simulink model "Base_Model"  (R2023b)
settings: Solver=VariableStepAuto  StartTime=0.0  StopTime=120  RelTol=1e-3
undefined symbols (not defined in the file): D1, D2, I
libraries: simulink x3, mcbcontrolslib x2
settings Model: Creator=markzhuang  LastModifiedBy=markzhuang

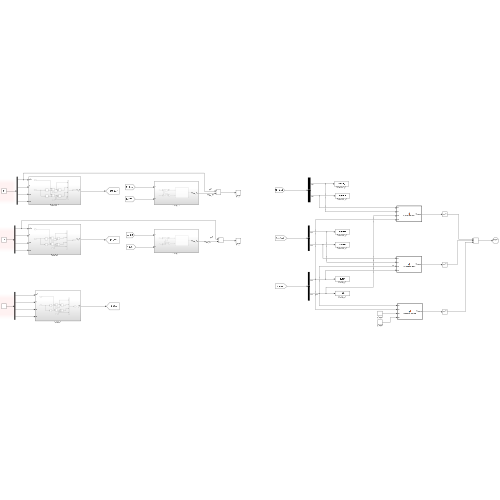
[thumbnail: Simulink's stored preview of the top-level diagram]
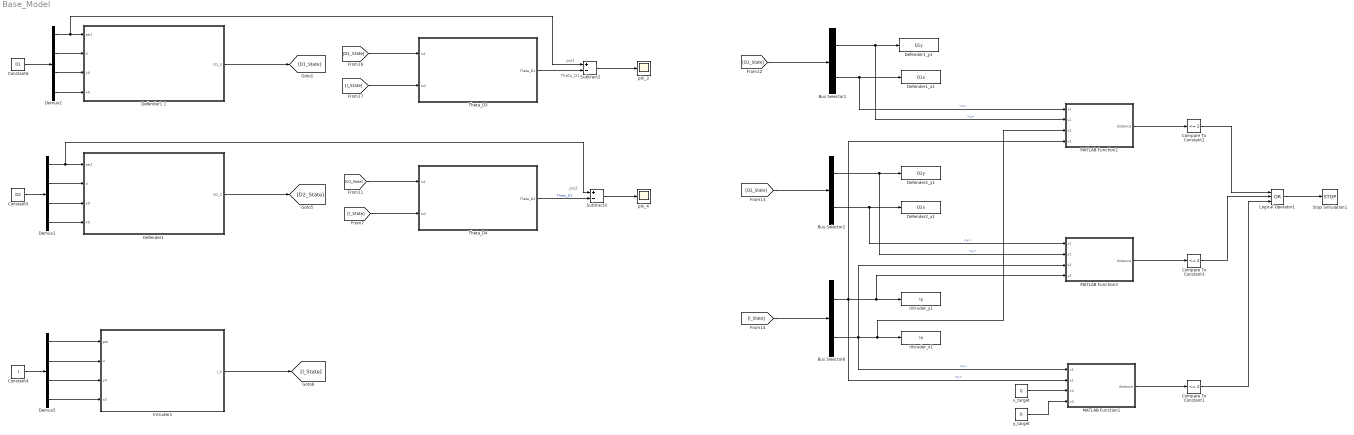
== system Base_Model ==
  note: psi2
  note: psi1
  note: Theta_D1
  Bus Selector1 : BusSelector  OutputSignals=y,x
  Bus Selector2 : BusSelector  OutputSignals=y,x
  Bus Selector6 : BusSelector  OutputSignals=y,x
  Compare To Constant1 : simulink/Logic and Bit Operations/Compare To Constant  relop=<=  const=2  OutDataTypeStr=boolean
  Compare To Constant2 : simulink/Logic and Bit Operations/Compare To Constant  relop=<=  const=2  OutDataTypeStr=boolean
  Compare To Constant3 : simulink/Logic and Bit Operations/Compare To Constant  relop=<=  const=2  OutDataTypeStr=boolean
  Constant4 : Constant  Value=I  VectorParams1D=off
  Constant5 : Constant  Value=D2  VectorParams1D=off
  Constant6 : Constant  Value=D1  VectorParams1D=off
  Defender1 : Subsystem
  Defender1 1 : Subsystem
  Defender1_x1 : ToWorkspace  VariableName=D1x  SaveFormat=Timeseries  SampleTime=-1
  Defender1_y1 : ToWorkspace  VariableName=D1y  SaveFormat=Timeseries  SampleTime=-1
  Defender2_x1 : ToWorkspace  VariableName=D2x  SaveFormat=Timeseries  SampleTime=-1
  Defender2_y1 : ToWorkspace  VariableName=D2y  SaveFormat=Timeseries  SampleTime=-1
  Demux1 : Demux
  Demux2 : Demux
  Demux5 : Demux
  Intruder1 : Subsystem
  Intruder_x1 : ToWorkspace  VariableName=Ix  SaveFormat=Timeseries  SampleTime=-1
  Intruder_y1 : ToWorkspace  VariableName=Iy  SaveFormat=Timeseries  SampleTime=-1
  Logical Operator1 : Logic  Operator=OR  Inputs=3  AllPortsSameDT=off  OutDataTypeStr=boolean
  MATLAB Function1 : MATLAB Function  TreatAsAtomicUnit=on
  MATLAB Function2 : MATLAB Function  TreatAsAtomicUnit=on
  MATLAB Function3 : MATLAB Function  TreatAsAtomicUnit=on
  Stop Simulation1 : Stop
  Subtract2 : Sum  Inputs=+-
  Subtract3 : Sum  Inputs=+-
  Theta_D3 : Subsystem
  Theta_D4 : Subsystem
  phi_3 : Scope
  phi_4 : Scope
  x_target : Constant  Value=0
  y_target : Constant  Value=0
  wires:
  Bus Selector1/2 -> MATLAB Function2/1(x1), Defender1_x1/1  "<x>"
  Demux5/3 -> Intruder1/3(y0)
  Demux5/4 -> Intruder1/4(x0)
  [D2_State] -> Theta_D4/1(In1)
  [D1_State] -> Theta_D3/1(In1)
  Bus Selector1/1 -> MATLAB Function2/2(y1), Defender1_y1/1  "<y>"
  Demux2/2 -> Defender1 1/2(V)
  y_target/1 -> MATLAB Function1/4(y2)
  Defender1 1/1(D1_S) -> [D1_State]
  Demux5/2 -> Intruder1/2(V)
  Demux2/3 -> Defender1 1/3(y0)
  Bus Selector6/1 -> MATLAB Function1/2(y1), MATLAB Function2/4(y2), MATLAB Function3/4(y2), Intruder_y1/1  "<y>"
  Demux5/1 -> Intruder1/1(psiI)
  Defender1/1(D2_S) -> [D2_State]
  [I_State] -> Theta_D3/2(In2)
  [I_State] -> Theta_D4/2(In2)
  Demux1/4 -> Defender1/4(x0)
  Constant6/1 -> Demux2/1
  MATLAB Function1/1(distance) -> Compare To Constant1/1
  Constant4/1 -> Demux5/1
  Demux1/2 -> Defender1/2(V)
  [D2_State] -> Bus Selector2/1
  Subtract2/1 -> phi_3/1
  MATLAB Function2/1(distance) -> Compare To Constant2/1
  MATLAB Function3/1(distance) -> Compare To Constant3/1
  Compare To Constant3/1 -> Logical Operator1/2
  Bus Selector2/1 -> MATLAB Function3/2(y1), Defender2_y1/1  "<y>"
  Demux1/3 -> Defender1/3(y0)
  Compare To Constant1/1 -> Logical Operator1/3
  Subtract3/1 -> phi_4/1
  Bus Selector2/2 -> MATLAB Function3/1(x1), Defender2_x1/1  "<x>"
  Demux2/4 -> Defender1 1/4(x0)
  Bus Selector6/2 -> MATLAB Function3/3(x2), MATLAB Function1/1(x1), MATLAB Function2/3(x2), Intruder_x1/1  "<x>"
  x_target/1 -> MATLAB Function1/3(x2)
  [D1_State] -> Bus Selector1/1
  Theta_D3/1(Theta_D1) -> Subtract2/2
  Logical Operator1/1 -> Stop Simulation1/1
  Compare To Constant2/1 -> Logical Operator1/1
  Intruder1/1(I_S) -> [I_State]
  Constant5/1 -> Demux1/1
  [I_State] -> Bus Selector6/1
  Theta_D4/1(Theta_D2) -> Subtract3/2  "Theta_D2"
  Demux2/1 -> Subtract2/1, Defender1 1/1(psi1)
  Demux1/1 -> Subtract3/1, Defender1/1(psi2)

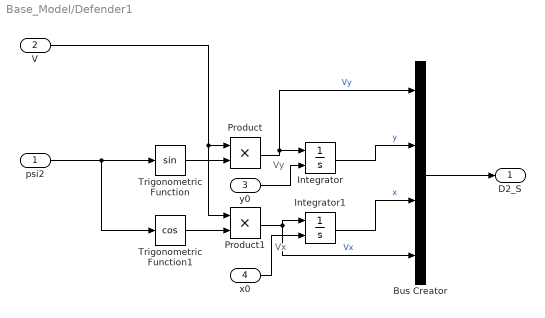
== system Base_Model/Defender1 ==
  note: Vx
  note: Vy
  psi2 : Inport
  V : Inport  Port=2
  y0 : Inport  Port=3
  x0 : Inport  Port=4
  Bus Creator : BusCreator  Inputs=4
  Integrator : Integrator  InitialConditionSource=external
  Integrator1 : Integrator  InitialConditionSource=external
  Product : Product
  Product1 : Product
  Trigonometric Function : Trigonometry
  Trigonometric Function1 : Trigonometry  Operator=cos
  D2_S : Outport
  wires:
  Trigonometric Function/1 -> Product/2
  Product/1 -> Bus Creator/1, Integrator/1  "Vy"
  psi2/1 -> Trigonometric Function1/1, Trigonometric Function/1
  Product1/1 -> Bus Creator/4, Integrator1/1  "Vx"
  V/1 -> Product1/1, Product/1
  Trigonometric Function1/1 -> Product1/2
  Integrator/1 -> Bus Creator/2  "y"
  Integrator1/1 -> Bus Creator/3  "x"
  y0/1 -> Integrator/2
  x0/1 -> Integrator1/2
  Bus Creator/1 -> D2_S/1

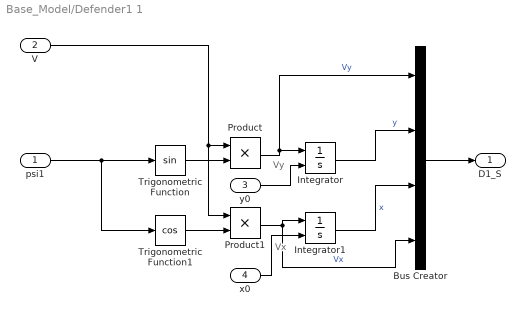
== system Base_Model/Defender1 1 ==
  note: Vx
  note: Vy
  psi1 : Inport
  V : Inport  Port=2
  y0 : Inport  Port=3
  x0 : Inport  Port=4
  Bus Creator : BusCreator  Inputs=4
  Integrator : Integrator  InitialConditionSource=external
  Integrator1 : Integrator  InitialConditionSource=external
  Product : Product
  Product1 : Product
  Trigonometric Function : Trigonometry
  Trigonometric Function1 : Trigonometry  Operator=cos
  D1_S : Outport
  wires:
  Trigonometric Function/1 -> Product/2
  psi1/1 -> Trigonometric Function1/1, Trigonometric Function/1
  Product1/1 -> Bus Creator/4, Integrator1/1  "Vx"
  V/1 -> Product1/1, Product/1
  Trigonometric Function1/1 -> Product1/2
  y0/1 -> Integrator/2
  x0/1 -> Integrator1/2
  Product/1 -> Bus Creator/1, Integrator/1  "Vy"
  Integrator/1 -> Bus Creator/2  "y"
  Integrator1/1 -> Bus Creator/3  "x"
  Bus Creator/1 -> D1_S/1

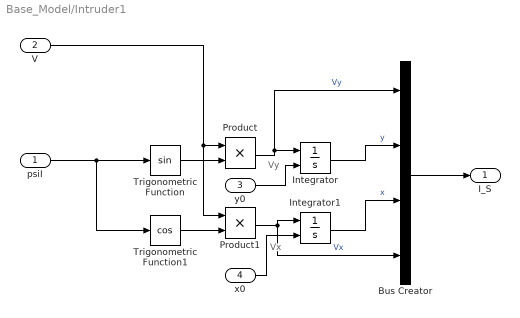
== system Base_Model/Intruder1 ==
  note: Vx
  note: Vy
  psiI : Inport
  V : Inport  Port=2
  y0 : Inport  Port=3
  x0 : Inport  Port=4
  Bus Creator : BusCreator  Inputs=4
  Integrator : Integrator  InitialConditionSource=external
  Integrator1 : Integrator  InitialConditionSource=external
  Product : Product
  Product1 : Product
  Trigonometric Function : Trigonometry
  Trigonometric Function1 : Trigonometry  Operator=cos
  I_S : Outport
  wires:
  Trigonometric Function/1 -> Product/2
  Product/1 -> Bus Creator/1, Integrator/1  "Vy"
  psiI/1 -> Trigonometric Function1/1, Trigonometric Function/1
  Product1/1 -> Bus Creator/4, Integrator1/1  "Vx"
  V/1 -> Product1/1, Product/1
  Trigonometric Function1/1 -> Product1/2
  Integrator/1 -> Bus Creator/2  "y"
  Integrator1/1 -> Bus Creator/3  "x"
  y0/1 -> Integrator/2
  x0/1 -> Integrator1/2
  Bus Creator/1 -> I_S/1

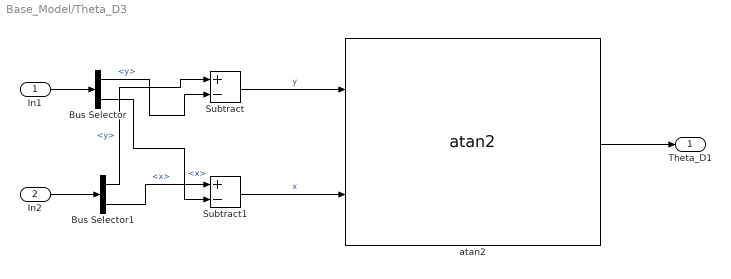
== system Base_Model/Theta_D3 ==
  In1 : Inport
  In2 : Inport  Port=2
  Bus Selector : BusSelector  OutputSignals=y,x
  Bus Selector1 : BusSelector  OutputSignals=y,x
  Subtract : Sum  Inputs=+-
  Subtract1 : Sum  Inputs=+-
  atan2 : mcbcontrolslib/atan2  ApproximationMethod=None  NumberOfIterations=11  NumberOfDataPoints=16  InterpMethod=Flat  outputUnit=Radians  TableDataTypeStr=Inherit: Inherit via input
      settings: LibrarySourceBlock=mcblib/Controls/Math Transforms/atan2
  Theta_D1 : Outport
  wires:
  In1/1 -> Bus Selector/1
  In2/1 -> Bus Selector1/1
  Bus Selector1/1 -> Subtract/1  "<y>"
  Bus Selector/1 -> Subtract/2  "<y>"
  Bus Selector1/2 -> Subtract1/1  "<x>"
  Bus Selector/2 -> Subtract1/2  "<x>"
  Subtract/1 -> atan2/1  "y"
  Subtract1/1 -> atan2/2  "x"
  atan2/1 -> Theta_D1/1

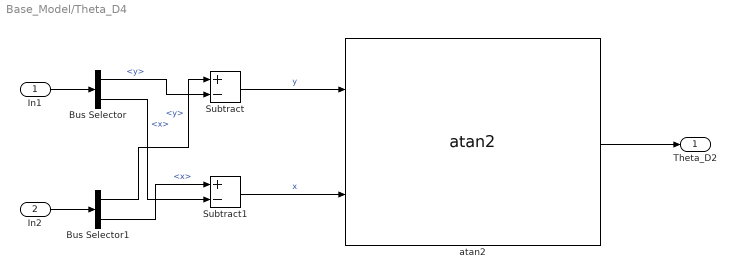
== system Base_Model/Theta_D4 ==
  In1 : Inport
  In2 : Inport  Port=2
  Bus Selector : BusSelector  OutputSignals=y,x
  Bus Selector1 : BusSelector  OutputSignals=y,x
  Subtract : Sum  Inputs=+-
  Subtract1 : Sum  Inputs=+-
  atan2 : mcbcontrolslib/atan2  ApproximationMethod=None  NumberOfIterations=11  NumberOfDataPoints=16  InterpMethod=Flat  outputUnit=Radians  TableDataTypeStr=Inherit: Inherit via input
      settings: LibrarySourceBlock=mcblib/Controls/Math Transforms/atan2
  Theta_D2 : Outport
  wires:
  In1/1 -> Bus Selector/1
  In2/1 -> Bus Selector1/1
  Bus Selector1/1 -> Subtract/1  "<y>"
  Bus Selector/1 -> Subtract/2  "<y>"
  Bus Selector1/2 -> Subtract1/1  "<x>"
  Bus Selector/2 -> Subtract1/2  "<x>"
  Subtract/1 -> atan2/1  "y"
  Subtract1/1 -> atan2/2  "x"
  atan2/1 -> Theta_D2/1

== matlab function Base_Model/MATLAB Function1 ==
  data: x1 input; distance output; y1 input; x2 input; y2 input
function distance = calculateDistance(x1, y1, x2, y2)
    distance = sqrt((x2 - x1)^2 + (y2 - y1)^2);
end

== matlab function Base_Model/MATLAB Function2 ==
  data: x1 input; distance output; y1 input; x2 input; y2 input
function distance = calculateDistance(x1, y1, x2, y2)
    distance = sqrt((x2 - x1)^2 + (y2 - y1)^2);
end

== matlab function Base_Model/MATLAB Function3 ==
  data: x1 input; distance output; y1 input; x2 input; y2 input
function distance = calculateDistance(x1, y1, x2, y2)
    distance = sqrt((x2 - x1)^2 + (y2 - y1)^2);
end
